simulink model "Quanser_AERO_Simulation_2020b"  (R2020b)
settings: Solver=ode45  StartTime=0.0  StopTime=sim_time  FixedStep=0.01  RelTol=1e-3
InitFcn:
  | % Run simulation parameters
  | quanser_AERO_sim_params;
model workspace (MAT data in the model file):
  a = Simulink.Parameter
  a.Value = 1.15
  a.DataType = 'auto'
  a.Dimensions = [1 1]
  a_a = Simulink.Parameter
  a_a.Value = 0.043381
  a_a.DataType = 'auto'
  a_a.Dimensions = [1 1]
  b = Simulink.Parameter
  b.Value = 0.2847
  b.DataType = 'auto'
  b.Dimensions = [1 1]
  b_b = Simulink.Parameter
  b_b.Value = 0.005
  b_b.DataType = 'auto'
  b_b.Dimensions = [1 1]
  c = Simulink.Parameter
  c.Value = 0.53573
  c.DataType = 'auto'
  c.Dimensions = [1 1]
  c_c = Simulink.Parameter
  c_c.Value = 0.005
  c_c.DataType = 'auto'
  c_c.Dimensions = [1 1]
  d = Simulink.Parameter
  d.Value = 0.0071058
  d.DataType = 'auto'
  d.Dimensions = [1 1]
  d_d = Simulink.Parameter
  d_d.Value = 0
  d_d.DataType = 'auto'
  d_d.Dimensions = [1 1]
  e = Simulink.Parameter
  e.Value = 0.0071
  e.DataType = 'auto'
  e.Dimensions = [1 1]
  f = Simulink.Parameter
  f.Value = 0.05
  f.DataType = 'auto'
  f.Dimensions = [1 1]
  g = Simulink.Parameter
  g.Value = 9.81
  g.DataType = 'auto'
  g.Dimensions = [1 1]
  p_p = Simulink.Parameter
  p_p.Value = 0.0005466
  p_p.DataType = 'auto'
  p_p.Dimensions = [1 1]
  smiData.RigidTransform(1).translation = [75 240 -4.4408920985e-15]
  smiData.RigidTransform(1).angle = 1.57079632679
  smiData.RigidTransform(1).axis = [5.55111512313e-17 1 5.55111512313e-17]
  smiData.RigidTransform(1).ID = 'B[AERO - Fork:1:-:AERO - Arm:1]'
  smiData.RigidTransform(2).translation = [0 0 72.5]
  smiData.RigidTransform(2).angle = 0
  smiData.RigidTransform(2).axis = [0 0 0]
  smiData.RigidTransform(2).ID = 'F[AERO - Fork:1:-:AERO - Arm:1]'
  smiData.RigidTransform(3).translation = [53 0 0]
  smiData.RigidTransform(3).angle = 1.57079632679
  smiData.RigidTransform(3).axis = [0 -1 0]
  smiData.RigidTransform(3).ID = 'B[AERO - Arm:1:-:AERO - Propeller Housing:1]'
  smiData.RigidTransform(4).translation = [-2.67952073108e-14 10 -95.5137103749]
  smiData.RigidTransform(4).angle = 3.14159265359
  smiData.RigidTransform(4).axis = [1 0 0]
  smiData.RigidTransform(4).ID = 'F[AERO - Arm:1:-:AERO - Propeller Housing:1]'
  smiData.RigidTransform(5).translation = [-53 0 0]
  smiData.RigidTransform(5).angle = 3.14159265359
  smiData.RigidTransform(5).axis = [0.707106781187 0 0.707106781187]
  smiData.RigidTransform(5).ID = 'B[AERO - Arm:1:-:AERO - Propeller Housing:2]'
  smiData.RigidTransform(6).translation = [-2.67952073108e-14 10 -95.5137103749]
  smiData.RigidTransform(6).angle = 3.14159265359
  smiData.RigidTransform(6).axis = [1 0 0]
  smiData.RigidTransform(6).ID = 'F[AERO - Arm:1:-:AERO - Propeller Housing:2]'
  smiData.RigidTransform(7).translation = [0 90 0]
  smiData.RigidTransform(7).angle = 2.09439510239
  smiData.RigidTransform(7).axis = [-0.57735026919 -0.57735026919 -0.57735026919]
  smiData.RigidTransform(7).ID = 'B[AERO - Base:1:-:AERO - Fork:1]'
  smiData.RigidTransform(8).translation = [0 -10 -1.83697019872e-15]
  smiData.RigidTransform(8).angle = 1.57079632679
  smiData.RigidTransform(8).axis = [-1 0 0]
  smiData.RigidTransform(8).ID = 'F[AERO - Base:1:-:AERO - Fork:1]'
  smiData.RigidTransform(9).translation = [0 7 0]
  smiData.RigidTransform(9).angle = 1.57079632679
  smiData.RigidTransform(9).axis = [-1 1.5327705937e-16 1.5327705937e-16]
  smiData.RigidTransform(9).ID = 'B[AERO - Propeller Housing:1:-:AERO - Propeller:1]'
  smiData.RigidTransform(10).translation = [0 2 0]
  smiData.RigidTransform(10).angle = 1.6664335536
  smiData.RigidTransform(10).axis = [-0.908660854566 0.295241808844 0.295241808844]
  smiData.RigidTransform(10).ID = 'F[AERO - Propeller Housing:1:-:AERO - Propeller:1]'
  smiData.RigidTransform(11).translation = [0 7 0]
  smiData.RigidTransform(11).angle = 1.57079632679
  smiData.RigidTransform(11).axis = [-1 6.25051204106e-17 6.25051204106e-17]
  smiData.RigidTransform(11).ID = 'B[AERO - Propeller Housing:2:-:AERO - Propeller:2]'
  smiData.RigidTransform(12).translation = [0 2 0]
  smiData.RigidTransform(12).angle = 2.28432867519
  smiData.RigidTransform(12).axis = [-0.456966311669 -0.628960169645 -0.628960169645]
  smiData.RigidTransform(12).ID = 'F[AERO - Propeller Housing:2:-:AERO - Propeller:2]'
  smiData.RigidTransform(13).translation = [-4.21383634609 -51.619496794 8.881784197e-15]
  smiData.RigidTransform(13).angle = 0
  smiData.RigidTransform(13).axis = [0 0 0]
  smiData.RigidTransform(13).ID = 'SixDofRigidTransform[AERO - Base:1]'
  smiData.Solid(1).mass = 2.36460135901
  smiData.Solid(1).CoM = [5.24111117378e-10 37.9532129776 0]
  smiData.Solid(1).MoI = [7187.732483 11870.3385044 7187.73246752]
  smiData.Solid(1).PoI = [0 0 -5.80827271444e-08]
  smiData.Solid(1).color = [0.0196078431373 0.0196078431373 0.0196078431373]
  smiData.Solid(1).opacity = 1
  smiData.Solid(1).ID = 'AERO - Base.ipt_{5B170AF7-4835-771C-6ADF-04BDBD784493}'
  smiData.Solid(2).mass = 0.833057949362
  smiData.Solid(2).CoM = [2.66169728603e-11 94.8876622043 1.47659785864e-12]
  smiData.Solid(2).MoI = [5303.1260885 5291.93963258 10383.1205417]
  smiData.Solid(2).PoI = [-1.78319566538e-10 1.20053300634e-10 2.21603950608e-09]
  smiData.Solid(2).color = [0.0196078431373 0.0196078431373 0.0196078431373]
  smiData.Solid(2).opacity = 1
  smiData.Solid(2).ID = 'AERO - Fork.ipt_{19DEB560-4DA8-F02E-E9C0-369FCF880C44}'
  smiData.Solid(3).mass = 0.268036846773
  smiData.Solid(3).CoM = [1.42171296006e-09 -5.19659809406e-10 0]
  smiData.Solid(3).MoI = [365.292105474 461.18513674 151.85502279]
  smiData.Solid(3).PoI = [9.09494701773e-14 -7.58518581279e-10 0]
  smiData.Solid(3).color = [0.0196078431373 0.0196078431373 0.0196078431373]
  smiData.Solid(3).opacity = 1
  smiData.Solid(3).ID = 'AERO - Arm.ipt_{15B1D815-460D-A329-2F9F-5FB9E93ED37B}'
  smiData.Solid(4).mass = 0.12383177107
  smiData.Solid(4).CoM = [0.00177195297055 5.45503898669 -8.60877968745]
  smiData.Solid(4).MoI = [310.701431452 411.715449483 138.600608927]
  smiData.Solid(4).PoI = [4.84491065682 -0.146839869659 -0.00100363322073]
  smiData.Solid(4).color = [0.0196078431373 0.0196078431373 0.0196078431373]
  smiData.Solid(4).opacity = 1
  smiData.Solid(4).ID = 'AERO - Propeller Housing.ipt_{180F9119-4C93-59E3-A88D-3BA97F46F3C3}'
  smiData.Solid(5).mass = 0.0206425497221
  smiData.Solid(5).CoM = [-1.0654070865e-12 5.09575570658 -2.10819251568e-11]
  smiData.Solid(5).MoI = [13.8216638961 27.2772869122 13.8216638974]
  smiData.Solid(5).PoI = [0 0 -9.39933149128e-14]
  smiData.Solid(5).color = [0.121568627451 0.121568627451 0.705882352941]
  smiData.Solid(5).opacity = 1
  smiData.Solid(5).ID = 'AERO - Propeller.ipt_{54ECD9B7-47A0-F6BB-CE8E-F5BB4731363E}'
  smiData.RevoluteJoint(1).Rz.Pos = 8.54433050095e-10
  smiData.RevoluteJoint(1).ID = '[AERO - Fork:1:-:AERO - Arm:1]'
  smiData.RevoluteJoint(2).Rz.Pos = 176.894023419
  smiData.RevoluteJoint(2).ID = '[AERO - Arm:1:-:AERO - Propeller Housing:1]'
  smiData.RevoluteJoint(3).Rz.Pos = 3.10597658118
  smiData.RevoluteJoint(3).ID = '[AERO - Arm:1:-:AERO - Propeller Housing:2]'
  smiData.RevoluteJoint(4).Rz.Pos = -4.73234748156e-11
  smiData.RevoluteJoint(4).ID = '[AERO - Base:1:-:AERO - Fork:1]'
  smiData.RevoluteJoint(5).Rz.Pos = -5.89066785065e-05
  smiData.RevoluteJoint(5).ID = '[AERO - Propeller Housing:1:-:AERO - Propeller:1]'
  smiData.RevoluteJoint(6).Rz.Pos = -3.64250166753e-05
  smiData.RevoluteJoint(6).ID = '[AERO - Propeller Housing:2:-:AERO - Propeller:2]'
  t_t = Simulink.Parameter
  t_t.Value = 0.0005466
  t_t.DataType = 'auto'
  t_t.Dimensions = [1 1]
  u_lim = Simulink.Parameter
  u_lim.Value = 24
  u_lim.DataType = 'auto'
  u_lim.Dimensions = [1 1]
  y_y = Simulink.Parameter
  y_y.Value = 0.02
  y_y.DataType = 'auto'
  y_y.Dimensions = [1 1]
  z_z = Simulink.Parameter
  z_z.Value = 0.01
  z_z.DataType = 'auto'
  z_z.Dimensions = [1 1]
undefined symbols (not defined in the file): A, A11, A12, A21, A22, A_tild, B, B1, B2, B_tild, C, C_tild, D_tild, ini_cond, Jr, KI, KII, KX, KXX, L, model, noise, ts, X, Y, Z
libraries: sm_lib x175, nesl_utility x35, simulink x30
(part 1 of 5)
settings Model: DataDictionary=AERO_DigitalTwin.sldd  OrderedModelArguments=off  Creator=garciar1  LastModifiedBy=linesLK

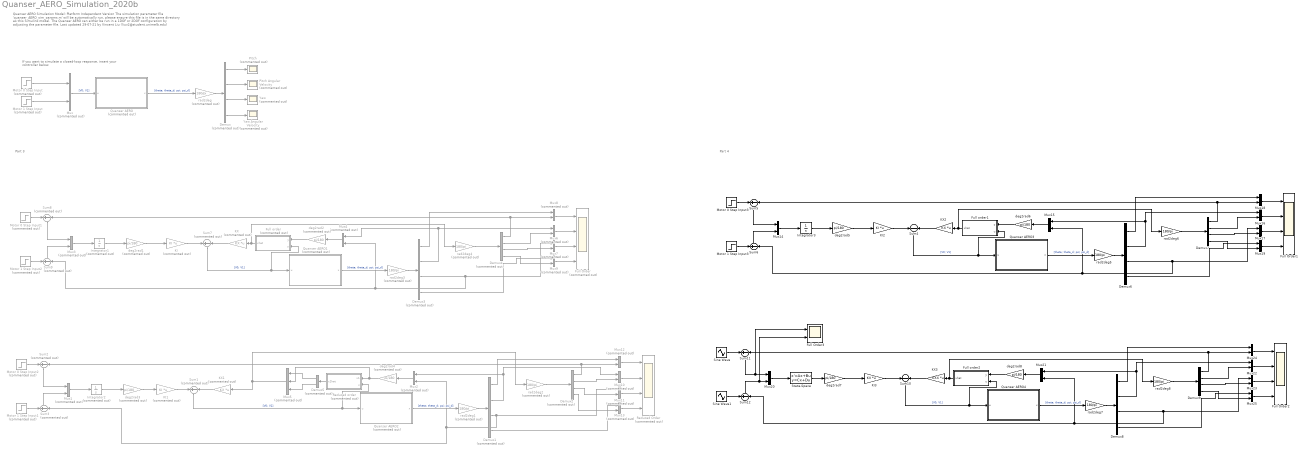
== system Quanser_AERO_Simulation_2020b ==
  note: If you want to simulate a closed-loop response, insert your controller below.
  note: Quanser AERO Simulation Model: Platform Independent Version
      | The simulation parameter file 'quanser_AERO_sim_params.m' will be automatically run, please ensure this file is in the same directory as this Simulink model. The Quanser AERO can either be run in a 1DOF or 2DOF configuration by adjusting the parameter file.
      | Last updated 29-07-21 by Vincent Liu (liuv2@student.unimelb.edu)
  note: Part 3
  note: Part 4
  Demux{,1..4} (5 alike) : Demux  Commented=on
  Demux5 : Demux  Commented=on  Outputs=2
  Demux{6..9} (4 alike) : Demux
  Full Order : Scope  Commented=on  NumInputPorts=4
  Full Order1 : Scope  NumInputPorts=4
  Full Order2 : Scope  NumInputPorts=4
  Full Order3 : Scope  NumInputPorts=2
  Full order : Subsystem  Commented=on
  Full order1 : Subsystem
  Full order2 : Subsystem
  Integrator1 : Integrator  Commented=on
  Integrator2 : Integrator  Commented=on
  Integrator3 : Integrator
  KI : Gain  Commented=on  Gain=KI  Multiplication=Matrix(K*u) (u vector)
  KI1 : Gain  Commented=on  Gain=KI  Multiplication=Matrix(K*u) (u vector)
  KI2 : Gain  Gain=KI  Multiplication=Matrix(K*u) (u vector)
  KI3 : Gain  Gain=KII  Multiplication=Matrix(K*u) (u vector)
  KX : Gain  Commented=on  Gain=KX  Multiplication=Matrix(K*u) (u vector)
  KX1 : Gain  Commented=on  Gain=KX  Multiplication=Matrix(K*u) (u vector)
  KX2 : Gain  Gain=KX  Multiplication=Matrix(K*u) (u vector)
  KX3 : Gain  Gain=KXX  Multiplication=Matrix(K*u) (u vector)
  Motor 0 Step Input : Step  Commented=on  After=20  SampleTime=0
  Motor 0 Step Input1 : Step  Commented=on  After=9  SampleTime=0
  Motor 0 Step Input2 : Step  Commented=on  After=9  SampleTime=0
  Motor 0 Step Input3 : Step  After=9  SampleTime=0
  Motor 1 Step Input : Step  Commented=on  After=10  SampleTime=0
  Motor 1 Step Input1 : Step  Commented=on  After=45  SampleTime=0
  Motor 1 Step Input2 : Step  Commented=on  After=45  SampleTime=0
  Motor 1 Step Input3 : Step  After=45  SampleTime=0
  Mux{,1..4,6..13} (13 alike) : Mux  Commented=on  Inputs=2
  Mux{14..25} (12 alike) : Mux  Inputs=2
  Mux5 : Mux  Commented=on  Inputs=3
  Pitch : Scope  Commented=on
  Pitch Angular Velocity : Scope  Commented=on
  Quanser AERO : Subsystem  Commented=on  TreatAsAtomicUnit=on
  Quanser AERO1 : Subsystem  Commented=on  TreatAsAtomicUnit=on
  Quanser AERO2 : Subsystem  Commented=on  TreatAsAtomicUnit=on
  Quanser AERO3 : Subsystem  TreatAsAtomicUnit=on
  Quanser AERO4 : Subsystem  TreatAsAtomicUnit=on
  Reduced Order : Scope  Commented=on  NumInputPorts=4
  Reduced order : Subsystem  Commented=on
  Sine Wave : Sin  Amplitude=9  Frequency=2*pi/5  SampleTime=0
  Sine Wave1 : Sin  Amplitude=30  Frequency=2*pi/5  SampleTime=0
  State-Space : StateSpace  A=A_tild  B=B_tild  C=C_tild  D=D_tild  InitialCondition=0
  Sum{1..3,7..9} (6 alike) : Sum  Commented=on  Inputs=+-
  Sum10 : Sum  Inputs=--
  Sum{5..6,11..12} (4 alike) : Sum  Inputs=+-
  Sum4 : Sum  Inputs=--
  Yaw : Scope  Commented=on
  Yaw Angular Velocity : Scope  Commented=on
  deg2rad{1..4} (4 alike) : Gain  Commented=on  Gain=pi/180
  deg2rad{5..8} (4 alike) : Gain  Gain=pi/180
  rad2deg{,1..4} (5 alike) : Gain  Commented=on  Gain=180/pi
  rad2deg{5..8} (4 alike) : Gain  Gain=180/pi
  wires:
  Demux/3 -> Yaw/1
  Demux/2 -> Pitch Angular Velocity/1
  Demux/4 -> Yaw Angular Velocity/1
  Mux/1 -> Quanser AERO/1(u)  "[V0; V1]"
  rad2deg/1 -> Demux/1
  Quanser AERO/1(x) -> rad2deg/1  "[theta; theta_d; psi; psi_d]"
  Motor 1 Step Input/1 -> Mux/2
  Motor 0 Step Input/1 -> Mux/1
  Demux/1 -> Pitch/1
  Mux3/1 -> Integrator1/1
  deg2rad1/1 -> KI/1
  Motor 1 Step Input2/1 -> Sum9/1
  Quanser AERO1/1(x) -> rad2deg3/1  "[theta; theta_d; psi; psi_d]"
  rad2deg3/1 -> Demux3/1
  KX/1 -> Sum7/2
  KI/1 -> Sum7/1
  Sum9/1 -> Mux3/2
  Sum7/1 -> Full order/2(u), Quanser AERO1/1(u)  "[V0; V1]"
  Integrator1/1 -> deg2rad1/1
  Motor 0 Step Input1/1 -> Sum8/1
  Sum8/1 -> Mux3/1
  Mux4/1 -> deg2rad2/1
  Full order/1(xhat) -> rad2deg4/1, KX/1
  deg2rad2/1 -> Full order/1(y)
  Demux4/3 -> Mux7/2
  rad2deg4/1 -> Demux4/1
  Demux3/2 -> Mux4/1, Mux6/1
  Demux4/2 -> Mux6/2
  Demux4/1 -> Mux8/2, Sum8/2
  Demux3/3 -> Mux7/1, Mux4/2, Sum9/2
  Sum2/1 -> Mux1/1
  KX1/1 -> Sum1/2
  Mux5/1 -> KX1/1, rad2deg2/1
  KI1/1 -> Sum1/1
  Quanser AERO2/1(x) -> rad2deg1/1  "[theta; theta_d; psi; psi_d]"
  Sum3/1 -> Mux1/2
  rad2deg2/1 -> Demux2/1
  Mux2/1 -> deg2rad4/1
  Motor 1 Step Input1/1 -> Sum3/1
  Motor 0 Step Input2/1 -> Sum2/1
  Sum1/1 -> Reduced order/2(u), Quanser AERO2/1(u)  "[V0; V1]"
  Demux1/3 -> Mux11/1, Mux2/2, Sum3/2
  Mux1/1 -> Integrator2/1
  deg2rad3/1 -> KI1/1
  Integrator2/1 -> deg2rad3/1
  rad2deg1/1 -> Demux1/1
  Demux2/1 -> Mux12/2, Sum2/2
  Demux1/2 -> Mux10/1, Mux2/1
  deg2rad4/1 -> Reduced order/1(x1), Mux5/2
  Reduced order/1(x2hat) -> Demux5/1
  Demux5/1 -> Mux5/1
  Demux5/2 -> Mux5/3
  Mux6/1 -> Full Order/2
  Mux7/1 -> Full Order/3
  Mux8/1 -> Full Order/1
  Demux3/1 -> Mux8/1
  Demux3/4 -> Mux9/1
  Demux4/4 -> Mux9/2
  Mux9/1 -> Full Order/4
  Mux13/1 -> Reduced Order/4
  Mux12/1 -> Reduced Order/1
  Mux11/1 -> Reduced Order/3
  Mux10/1 -> Reduced Order/2
  Demux1/1 -> Mux12/1
  Demux2/2 -> Mux10/2
  Demux2/3 -> Mux11/2
  Demux1/4 -> Mux13/1
  Demux2/4 -> Mux13/2
  deg2rad5/1 -> KI2/1
  Sum6/1 -> Mux14/2
  Demux7/4 -> Mux19/2
  Motor 0 Step Input3/1 -> Sum5/1
  Mux17/1 -> Full Order1/3
  Demux6/2 -> Mux16/1, Mux15/1
  Demux7/2 -> Mux16/2
  KI2/1 -> Sum4/1
  Quanser AERO3/1(x) -> rad2deg5/1  "[theta; theta_d; psi; psi_d]"
  KX2/1 -> Sum4/2
  deg2rad6/1 -> Full order1/1(y)
  Mux15/1 -> deg2rad6/1
  rad2deg6/1 -> Demux7/1
  Full order1/1(xhat) -> rad2deg6/1, KX2/1
  Demux6/1 -> Mux18/1
  rad2deg5/1 -> Demux6/1
  Sum4/1 -> Full order1/2(u), Quanser AERO3/1(u)  "[V0; V1]"
  Integrator3/1 -> deg2rad5/1
  Demux6/3 -> Mux17/1, Mux15/2, Sum6/2
  Mux14/1 -> Integrator3/1
  Mux18/1 -> Full Order1/1
  Motor 1 Step Input3/1 -> Sum6/1
  Mux16/1 -> Full Order1/2
  Sum5/1 -> Mux14/1
  Demux7/1 -> Mux18/2, Sum5/2
  Mux19/1 -> Full Order1/4
  Demux6/4 -> Mux19/1
  Demux7/3 -> Mux17/2
  Sum10/1 -> Full order2/2(u), Quanser AERO4/1(u)  "[V0; V1]"
  Sine Wave/1 -> Sum11/1
  Quanser AERO4/1(x) -> rad2deg7/1  "[theta; theta_d; psi; psi_d]"
  Demux9/3 -> Mux23/2
  deg2rad7/1 -> KI3/1
  rad2deg8/1 -> Demux9/1
  Demux9/4 -> Mux25/2
  Sum11/1 -> Full Order3/1, Mux20/1
  Mux20/1 -> State-Space/1
  KX3/1 -> Sum10/2
  Mux21/1 -> deg2rad8/1
  rad2deg7/1 -> Demux8/1
  Demux8/3 -> Mux23/1, Mux21/2, Sum12/2
  State-Space/1 -> deg2rad7/1
  deg2rad8/1 -> Full order2/1(y)
  Demux8/1 -> Mux24/1
  Sine Wave1/1 -> Sum12/1
  Demux8/2 -> Mux22/1, Mux21/1
  Mux22/1 -> Full Order2/2
  Mux24/1 -> Full Order2/1
  Demux9/1 -> Mux24/2, Sum11/2
  Mux25/1 -> Full Order2/4
  Demux9/2 -> Mux22/2
  Full order2/1(xhat) -> rad2deg8/1, KX3/1
  Demux8/4 -> Mux25/1
  Mux23/1 -> Full Order2/3
  KI3/1 -> Sum10/1
  Sum12/1 -> Full Order3/2, Mux20/2

== system Quanser_AERO_Simulation_2020b/Full order ==
  y : Inport
  u : Inport  Port=2
  A : Gain  Gain=A  Multiplication=Matrix(K*u) (u vector)
  B : Gain  Gain=B  Multiplication=Matrix(K*u) (u vector)
  C : Gain  Gain=C  Multiplication=Matrix(K*u) (u vector)
  Integrator1 : Integrator
  L : Gain  Gain=L  Multiplication=Matrix(K*u) (u vector)
  Sum1 : Sum  Inputs=+++
  Sum7 : Sum  Inputs=+-
  xhat : Outport
  wires:
  u/1 -> B/1
  Sum1/1 -> Integrator1/1
  y/1 -> Sum7/1
  C/1 -> Sum7/2
  Sum7/1 -> L/1
  L/1 -> Sum1/1
  B/1 -> Sum1/2
  A/1 -> Sum1/3
  Integrator1/1 -> C/1, A/1, xhat/1

== system Quanser_AERO_Simulation_2020b/Full order1 ==
  y : Inport
  u : Inport  Port=2
  A : Gain  Gain=A  Multiplication=Matrix(K*u) (u vector)
  B : Gain  Gain=B  Multiplication=Matrix(K*u) (u vector)
  C : Gain  Gain=C  Multiplication=Matrix(K*u) (u vector)
  Integrator1 : Integrator
  L : Gain  Gain=L  Multiplication=Matrix(K*u) (u vector)
  Sum1 : Sum  Inputs=+++
  Sum7 : Sum  Inputs=+-
  xhat : Outport
  wires:
  u/1 -> B/1
  Sum1/1 -> Integrator1/1
  y/1 -> Sum7/1
  C/1 -> Sum7/2
  Sum7/1 -> L/1
  L/1 -> Sum1/1
  B/1 -> Sum1/2
  A/1 -> Sum1/3
  Integrator1/1 -> C/1, A/1, xhat/1

== system Quanser_AERO_Simulation_2020b/Full order2 ==
  y : Inport
  u : Inport  Port=2
  A : Gain  Gain=A  Multiplication=Matrix(K*u) (u vector)
  B : Gain  Gain=B  Multiplication=Matrix(K*u) (u vector)
  C : Gain  Gain=C  Multiplication=Matrix(K*u) (u vector)
  Integrator1 : Integrator
  L : Gain  Gain=L  Multiplication=Matrix(K*u) (u vector)
  Sum1 : Sum  Inputs=+++
  Sum7 : Sum  Inputs=+-
  xhat : Outport
  wires:
  u/1 -> B/1
  Sum1/1 -> Integrator1/1
  y/1 -> Sum7/1
  C/1 -> Sum7/2
  Sum7/1 -> L/1
  L/1 -> Sum1/1
  B/1 -> Sum1/2
  A/1 -> Sum1/3
  Integrator1/1 -> C/1, A/1, xhat/1

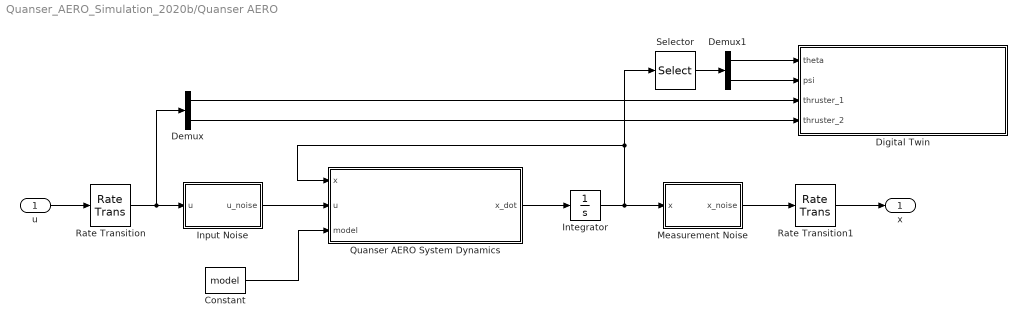
== system Quanser_AERO_Simulation_2020b/Quanser AERO ==
  u : Inport
  Constant : Constant  Value=model
  Demux : Demux  Outputs=2
  Demux1 : Demux  Outputs=2
  Digital Twin : Subsystem
  Input Noise : Subsystem  TreatAsAtomicUnit=on
  Integrator : Integrator  InitialCondition=[ini_cond.theta; ini_cond.theta_dot; ini_cond.psi; ini_cond.psi_dot]
  Measurement Noise : Subsystem  TreatAsAtomicUnit=on
  Quanser AERO System Dynamics : Subsystem  TreatAsAtomicUnit=on
  Rate Transition : RateTransition  OutPortSampleTime=ts
  Rate Transition1 : RateTransition  InitialCondition=[ini_cond.theta; ini_cond.theta_dot; ini_cond.psi; ini_cond.psi_dot]  OutPortSampleTime=ts
  Selector : Selector  InputPortWidth=4  IndexOptions=Index vector (dialog)  Indices=[1 3]  OutputSizes=1
  x : Outport  VectorParamsAs1DForOutWhenUnconnected=off
  wires:
  u/1 -> Rate Transition/1
  Rate Transition/1 -> Input Noise/1(u), Demux/1
  Rate Transition1/1 -> x/1
  Input Noise/1(u_noise) -> Quanser AERO System Dynamics/2(u)
  Measurement Noise/1(x_noise) -> Rate Transition1/1
  Selector/1 -> Demux1/1
  Demux/1 -> Digital Twin/3(thruster_1)
  Demux/2 -> Digital Twin/4(thruster_2)
  Demux1/1 -> Digital Twin/1(theta)
  Demux1/2 -> Digital Twin/2(psi)
  Integrator/1 -> Measurement Noise/1(x), Selector/1, Quanser AERO System Dynamics/1(x)
  Constant/1 -> Quanser AERO System Dynamics/3(model)
  Quanser AERO System Dynamics/1(x_dot) -> Integrator/1

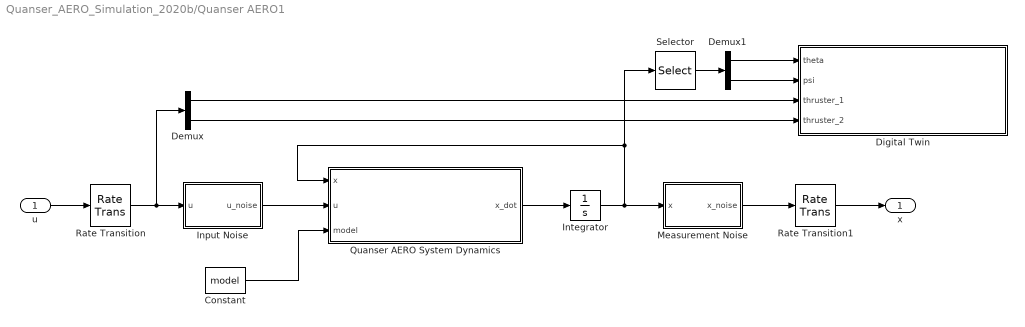
== system Quanser_AERO_Simulation_2020b/Quanser AERO1 ==
  u : Inport
  Constant : Constant  Value=model
  Demux : Demux  Outputs=2
  Demux1 : Demux  Outputs=2
  Digital Twin : Subsystem
  Input Noise : Subsystem  TreatAsAtomicUnit=on
  Integrator : Integrator  InitialCondition=[ini_cond.theta; ini_cond.theta_dot; ini_cond.psi; ini_cond.psi_dot]
  Measurement Noise : Subsystem  TreatAsAtomicUnit=on
  Quanser AERO System Dynamics : Subsystem  TreatAsAtomicUnit=on
  Rate Transition : RateTransition  OutPortSampleTime=ts
  Rate Transition1 : RateTransition  InitialCondition=[ini_cond.theta; ini_cond.theta_dot; ini_cond.psi; ini_cond.psi_dot]  OutPortSampleTime=ts
  Selector : Selector  InputPortWidth=4  IndexOptions=Index vector (dialog)  Indices=[1 3]  OutputSizes=1
  x : Outport  VectorParamsAs1DForOutWhenUnconnected=off
  wires:
  u/1 -> Rate Transition/1
  Rate Transition/1 -> Input Noise/1(u), Demux/1
  Rate Transition1/1 -> x/1
  Input Noise/1(u_noise) -> Quanser AERO System Dynamics/2(u)
  Measurement Noise/1(x_noise) -> Rate Transition1/1
  Selector/1 -> Demux1/1
  Demux/1 -> Digital Twin/3(thruster_1)
  Demux/2 -> Digital Twin/4(thruster_2)
  Demux1/1 -> Digital Twin/1(theta)
  Demux1/2 -> Digital Twin/2(psi)
  Integrator/1 -> Measurement Noise/1(x), Selector/1, Quanser AERO System Dynamics/1(x)
  Constant/1 -> Quanser AERO System Dynamics/3(model)
  Quanser AERO System Dynamics/1(x_dot) -> Integrator/1

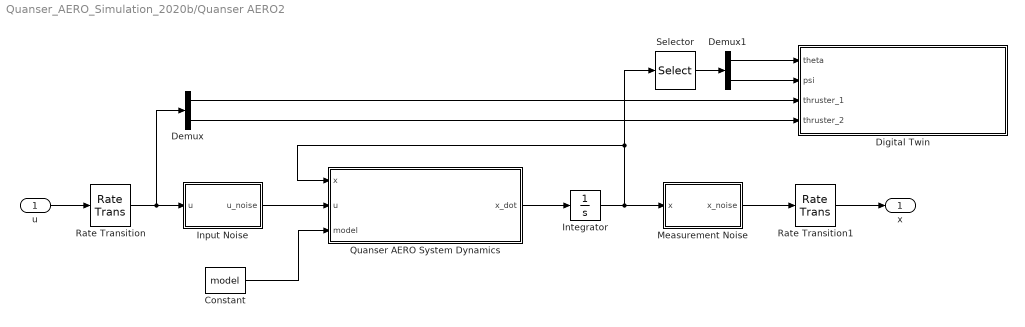
== system Quanser_AERO_Simulation_2020b/Quanser AERO2 ==
  u : Inport
  Constant : Constant  Value=model
  Demux : Demux  Outputs=2
  Demux1 : Demux  Outputs=2
  Digital Twin : Subsystem
  Input Noise : Subsystem  TreatAsAtomicUnit=on
  Integrator : Integrator  InitialCondition=[ini_cond.theta; ini_cond.theta_dot; ini_cond.psi; ini_cond.psi_dot]
  Measurement Noise : Subsystem  TreatAsAtomicUnit=on
  Quanser AERO System Dynamics : Subsystem  TreatAsAtomicUnit=on
  Rate Transition : RateTransition  OutPortSampleTime=ts
  Rate Transition1 : RateTransition  InitialCondition=[ini_cond.theta; ini_cond.theta_dot; ini_cond.psi; ini_cond.psi_dot]  OutPortSampleTime=ts
  Selector : Selector  InputPortWidth=4  IndexOptions=Index vector (dialog)  Indices=[1 3]  OutputSizes=1
  x : Outport  VectorParamsAs1DForOutWhenUnconnected=off
  wires:
  u/1 -> Rate Transition/1
  Rate Transition/1 -> Input Noise/1(u), Demux/1
  Rate Transition1/1 -> x/1
  Input Noise/1(u_noise) -> Quanser AERO System Dynamics/2(u)
  Measurement Noise/1(x_noise) -> Rate Transition1/1
  Selector/1 -> Demux1/1
  Demux/1 -> Digital Twin/3(thruster_1)
  Demux/2 -> Digital Twin/4(thruster_2)
  Demux1/1 -> Digital Twin/1(theta)
  Demux1/2 -> Digital Twin/2(psi)
  Integrator/1 -> Measurement Noise/1(x), Selector/1, Quanser AERO System Dynamics/1(x)
  Constant/1 -> Quanser AERO System Dynamics/3(model)
  Quanser AERO System Dynamics/1(x_dot) -> Integrator/1

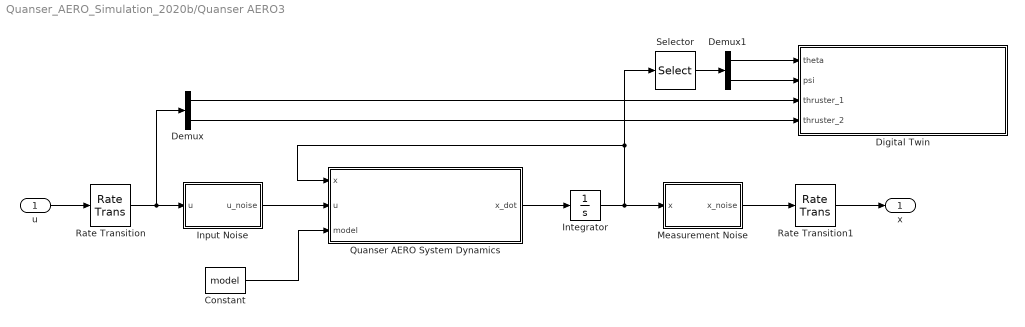
== system Quanser_AERO_Simulation_2020b/Quanser AERO3 ==
  u : Inport
  Constant : Constant  Value=model
  Demux : Demux  Outputs=2
  Demux1 : Demux  Outputs=2
  Digital Twin : Subsystem
  Input Noise : Subsystem  TreatAsAtomicUnit=on
  Integrator : Integrator  InitialCondition=[ini_cond.theta; ini_cond.theta_dot; ini_cond.psi; ini_cond.psi_dot]
  Measurement Noise : Subsystem  TreatAsAtomicUnit=on
  Quanser AERO System Dynamics : Subsystem  TreatAsAtomicUnit=on
  Rate Transition : RateTransition  OutPortSampleTime=ts
  Rate Transition1 : RateTransition  InitialCondition=[ini_cond.theta; ini_cond.theta_dot; ini_cond.psi; ini_cond.psi_dot]  OutPortSampleTime=ts
  Selector : Selector  InputPortWidth=4  IndexOptions=Index vector (dialog)  Indices=[1 3]  OutputSizes=1
  x : Outport  VectorParamsAs1DForOutWhenUnconnected=off
  wires:
  u/1 -> Rate Transition/1
  Rate Transition/1 -> Input Noise/1(u), Demux/1
  Rate Transition1/1 -> x/1
  Input Noise/1(u_noise) -> Quanser AERO System Dynamics/2(u)
  Measurement Noise/1(x_noise) -> Rate Transition1/1
  Selector/1 -> Demux1/1
  Demux/1 -> Digital Twin/3(thruster_1)
  Demux/2 -> Digital Twin/4(thruster_2)
  Demux1/1 -> Digital Twin/1(theta)
  Demux1/2 -> Digital Twin/2(psi)
  Integrator/1 -> Measurement Noise/1(x), Selector/1, Quanser AERO System Dynamics/1(x)
  Constant/1 -> Quanser AERO System Dynamics/3(model)
  Quanser AERO System Dynamics/1(x_dot) -> Integrator/1

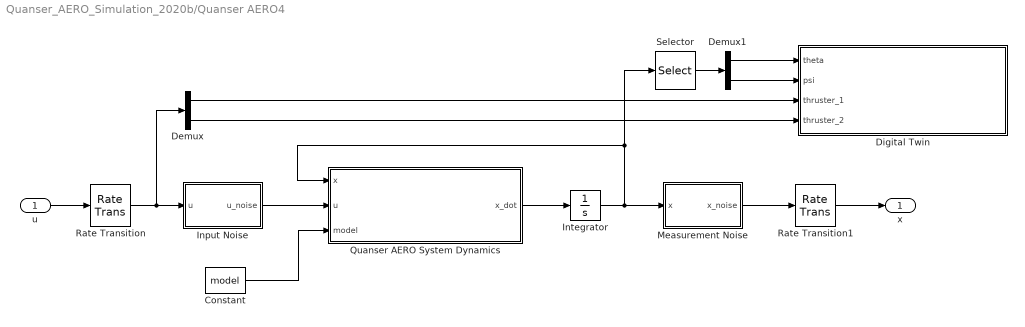
== system Quanser_AERO_Simulation_2020b/Quanser AERO4 ==
  u : Inport
  Constant : Constant  Value=model
  Demux : Demux  Outputs=2
  Demux1 : Demux  Outputs=2
  Digital Twin : Subsystem
  Input Noise : Subsystem  TreatAsAtomicUnit=on
  Integrator : Integrator  InitialCondition=[ini_cond.theta; ini_cond.theta_dot; ini_cond.psi; ini_cond.psi_dot]
  Measurement Noise : Subsystem  TreatAsAtomicUnit=on
  Quanser AERO System Dynamics : Subsystem  TreatAsAtomicUnit=on
  Rate Transition : RateTransition  OutPortSampleTime=ts
  Rate Transition1 : RateTransition  InitialCondition=[ini_cond.theta; ini_cond.theta_dot; ini_cond.psi; ini_cond.psi_dot]  OutPortSampleTime=ts
  Selector : Selector  InputPortWidth=4  IndexOptions=Index vector (dialog)  Indices=[1 3]  OutputSizes=1
  x : Outport  VectorParamsAs1DForOutWhenUnconnected=off
  wires:
  u/1 -> Rate Transition/1
  Rate Transition/1 -> Input Noise/1(u), Demux/1
  Rate Transition1/1 -> x/1
  Input Noise/1(u_noise) -> Quanser AERO System Dynamics/2(u)
  Measurement Noise/1(x_noise) -> Rate Transition1/1
  Selector/1 -> Demux1/1
  Demux/1 -> Digital Twin/3(thruster_1)
  Demux/2 -> Digital Twin/4(thruster_2)
  Demux1/1 -> Digital Twin/1(theta)
  Demux1/2 -> Digital Twin/2(psi)
  Integrator/1 -> Measurement Noise/1(x), Selector/1, Quanser AERO System Dynamics/1(x)
  Constant/1 -> Quanser AERO System Dynamics/3(model)
  Quanser AERO System Dynamics/1(x_dot) -> Integrator/1

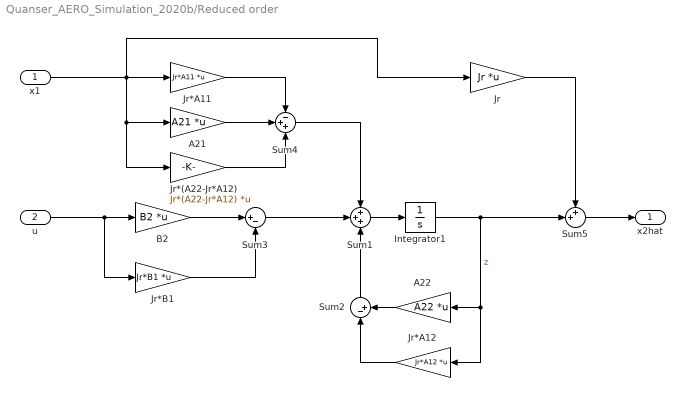
== system Quanser_AERO_Simulation_2020b/Reduced order ==
  x1 : Inport
  u : Inport  Port=2
  A21 : Gain  Gain=A21  Multiplication=Matrix(K*u) (u vector)
  A22 : Gain  Gain=A22  Multiplication=Matrix(K*u) (u vector)
  B2 : Gain  Gain=B2  Multiplication=Matrix(K*u) (u vector)
  Integrator1 : Integrator
  Jr : Gain  Gain=Jr  Multiplication=Matrix(K*u) (u vector)
  Jr*(A22-Jr*A12) : Gain  Gain=Jr*(A22-Jr*A12)  Multiplication=Matrix(K*u) (u vector)
  Jr*A11 : Gain  Gain=Jr*A11  Multiplication=Matrix(K*u) (u vector)
  Jr*A12 : Gain  Gain=Jr*A12  Multiplication=Matrix(K*u) (u vector)
  Jr*B1 : Gain  Gain=Jr*B1  Multiplication=Matrix(K*u) (u vector)
  Sum1 : Sum  Inputs=+++
  Sum2 : Sum  Inputs=|-+
  Sum3 : Sum  Inputs=|+-
  Sum4 : Sum  Inputs=-++
  Sum5 : Sum  Inputs=++|
  x2hat : Outport
  wires:
  Jr/1 -> Sum5/1
  B2/1 -> Sum3/1
  Sum4/1 -> Sum1/1
  Sum1/1 -> Integrator1/1
  Sum5/1 -> x2hat/1
  Sum2/1 -> Sum1/3
  Integrator1/1 -> Sum5/2, Jr*A12/1, A22/1  "z"
  Jr*A12/1 -> Sum2/1
  A21/1 -> Sum4/2
  Jr*A11/1 -> Sum4/1
  A22/1 -> Sum2/2
  x1/1 -> Jr*(A22-Jr*A12)/1, A21/1, Jr/1, Jr*A11/1
  u/1 -> Jr*B1/1, B2/1
  Jr*B1/1 -> Sum3/2
  Sum3/1 -> Sum1/2
  Jr*(A22-Jr*A12)/1 -> Sum4/3

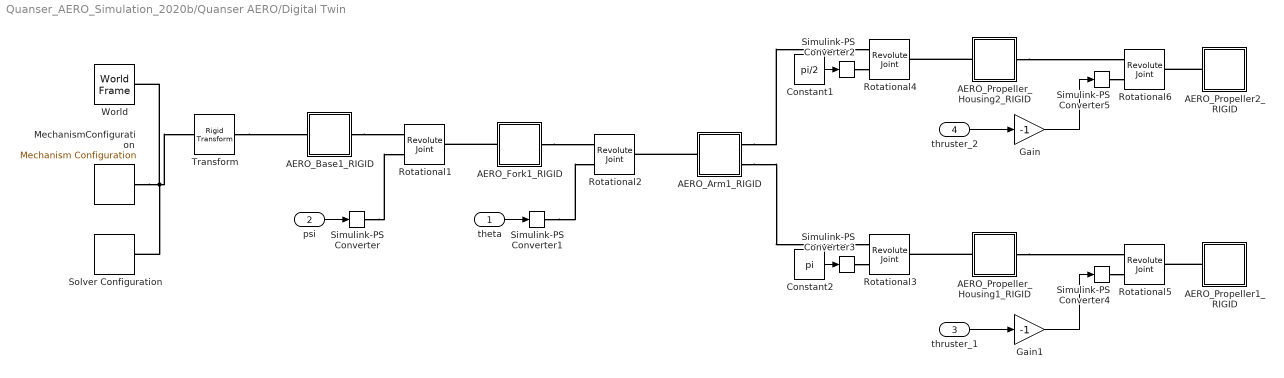
== system Quanser_AERO_Simulation_2020b/Quanser AERO/Digital Twin ==
  theta : Inport
  psi : Inport  Port=2
  thruster_1 : Inport  Port=3
  thruster_2 : Inport  Port=4
  AERO_Arm1_RIGID : Subsystem
  AERO_Base1_RIGID : Subsystem
  AERO_Fork1_RIGID : Subsystem
  AERO_Propeller1_RIGID : Subsystem
  AERO_Propeller2_RIGID : Subsystem
  AERO_Propeller_Housing1_RIGID : Subsystem
  AERO_Propeller_Housing2_RIGID : Subsystem
  Constant1 : Constant  Value=pi/2
  Constant2 : Constant  Value=pi
  Gain : Gain  Gain=-1
  Gain1 : Gain  Gain=-1
  MechanismConfiguration : sm_lib/Utilities/Mechanism Configuration  UniformGravity=Constant  GravityVector=[0 -9.80665 0]  GravityVectorUnits=m/s^2  GravityUnits=m/s^2  LinearizationDelta=0.001  JointModeTransitionNonlinearIterations=2
  Rotational1 : sm_lib/Joints/Revolute Joint  JointMode=Normal  SenseConstraintForce=off  SenseConstraintForceX=off  SenseConstraintForceY=off  SenseConstraintForceZ=off  SenseConstraintTorque=off  SenseConstraintTorqueX=off  SenseConstraintTorqueY=off  SenseConstraintTorqueZ=off  SenseTotalForce=off  SenseTotalForceX=off  SenseTotalForceY=off  SenseTotalForceZ=off  SenseTotalTorque=off  SenseTotalTorqueX=off  SenseTotalTorqueY=off  SenseTotalTorqueZ=off  CompositeWrenchDir=FollowerOnBase  CompositeWrenchFrame=BaseFrame  EquilibriumPosition=0  EquilibriumPositionUnits=deg  SpringStiffness=0  SpringStiffnessUnits=N*m/deg  DampingCoefficient=0  DampingCoefficientUnits=N*m/(deg/s)  TorqueActuationMode=ComputedTorque  MotionActuationMode=InputMotion  SensePosition=off  SenseVelocity=off  SenseAcceleration=off  SenseTorqueForce=off  SenseLowerLimitTorqueForce=off  SenseUpperLimitTorqueForce=off  LowerLimitSpecify=off  LowerLimitBound=-90  LowerLimitBoundUnits=deg  LowerLimitStiffness=1e4  LowerLimitStiffnessUnits=N*m/deg  LowerLimitDamping=10  LowerLimitDampingUnits=N*m/(deg/s)  LowerLimitTransitionRegionWidth=0.1  LowerLimitTransitionRegionWidthUnits=deg  UpperLimitSpecify=off  UpperLimitBound=90  UpperLimitBoundUnits=deg  UpperLimitStiffness=1e4  UpperLimitStiffnessUnits=N*m/deg  UpperLimitDamping=10  UpperLimitDampingUnits=N*m/(deg/s)  UpperLimitTransitionRegionWidth=0.1  UpperLimitTransitionRegionWidthUnits=deg  PositionTargetSpecify=on  PositionTargetPriority=Low  PositionTargetValue=smiData.RevoluteJoint(4).Rz.Pos  PositionTargetValueUnits=deg  VelocityTargetSpecify=off  VelocityTargetPriority=High  VelocityTargetValue=0  VelocityTargetValueUnits=deg/s
  Rotational2 : sm_lib/Joints/Revolute Joint  JointMode=Normal  SenseConstraintForce=off  SenseConstraintForceX=off  SenseConstraintForceY=off  SenseConstraintForceZ=off  SenseConstraintTorque=off  SenseConstraintTorqueX=off  SenseConstraintTorqueY=off  SenseConstraintTorqueZ=off  SenseTotalForce=off  SenseTotalForceX=off  SenseTotalForceY=off  SenseTotalForceZ=off  SenseTotalTorque=off  SenseTotalTorqueX=off  SenseTotalTorqueY=off  SenseTotalTorqueZ=off  CompositeWrenchDir=FollowerOnBase  CompositeWrenchFrame=BaseFrame  EquilibriumPosition=0  EquilibriumPositionUnits=deg  SpringStiffness=0  SpringStiffnessUnits=N*m/deg  DampingCoefficient=0  DampingCoefficientUnits=N*m/(deg/s)  TorqueActuationMode=ComputedTorque  MotionActuationMode=InputMotion  SensePosition=off  SenseVelocity=off  SenseAcceleration=off  SenseTorqueForce=off  SenseLowerLimitTorqueForce=off  SenseUpperLimitTorqueForce=off  LowerLimitSpecify=off  LowerLimitBound=-90  LowerLimitBoundUnits=deg  LowerLimitStiffness=1e4  LowerLimitStiffnessUnits=N*m/deg  LowerLimitDamping=10  LowerLimitDampingUnits=N*m/(deg/s)  LowerLimitTransitionRegionWidth=0.1  LowerLimitTransitionRegionWidthUnits=deg  UpperLimitSpecify=off  UpperLimitBound=90  UpperLimitBoundUnits=deg  UpperLimitStiffness=1e4  UpperLimitStiffnessUnits=N*m/deg  UpperLimitDamping=10  UpperLimitDampingUnits=N*m/(deg/s)  UpperLimitTransitionRegionWidth=0.1  UpperLimitTransitionRegionWidthUnits=deg  PositionTargetSpecify=on  PositionTargetPriority=Low  PositionTargetValue=smiData.RevoluteJoint(1).Rz.Pos  PositionTargetValueUnits=deg  VelocityTargetSpecify=off  VelocityTargetPriority=High  VelocityTargetValue=0  VelocityTargetValueUnits=deg/s
  Rotational3 : sm_lib/Joints/Revolute Joint  JointMode=Normal  SenseConstraintForce=off  SenseConstraintForceX=off  SenseConstraintForceY=off  SenseConstraintForceZ=off  SenseConstraintTorque=off  SenseConstraintTorqueX=off  SenseConstraintTorqueY=off  SenseConstraintTorqueZ=off  SenseTotalForce=off  SenseTotalForceX=off  SenseTotalForceY=off  SenseTotalForceZ=off  SenseTotalTorque=off  SenseTotalTorqueX=off  SenseTotalTorqueY=off  SenseTotalTorqueZ=off  CompositeWrenchDir=FollowerOnBase  CompositeWrenchFrame=BaseFrame  EquilibriumPosition=0  EquilibriumPositionUnits=deg  SpringStiffness=0  SpringStiffnessUnits=N*m/deg  DampingCoefficient=0  DampingCoefficientUnits=N*m/(deg/s)  TorqueActuationMode=ComputedTorque  MotionActuationMode=InputMotion  SensePosition=off  SenseVelocity=off  SenseAcceleration=off  SenseTorqueForce=off  SenseLowerLimitTorqueForce=off  SenseUpperLimitTorqueForce=off  LowerLimitSpecify=off  LowerLimitBound=-90  LowerLimitBoundUnits=deg  LowerLimitStiffness=1e4  LowerLimitStiffnessUnits=N*m/deg  LowerLimitDamping=10  LowerLimitDampingUnits=N*m/(deg/s)  LowerLimitTransitionRegionWidth=0.1  LowerLimitTransitionRegionWidthUnits=deg  UpperLimitSpecify=off  UpperLimitBound=90  UpperLimitBoundUnits=deg  UpperLimitStiffness=1e4  UpperLimitStiffnessUnits=N*m/deg  UpperLimitDamping=10  UpperLimitDampingUnits=N*m/(deg/s)  UpperLimitTransitionRegionWidth=0.1  UpperLimitTransitionRegionWidthUnits=deg  PositionTargetSpecify=on  PositionTargetPriority=High  PositionTargetValue=smiData.RevoluteJoint(2).Rz.Pos  PositionTargetValueUnits=deg  VelocityTargetSpecify=off  VelocityTargetPriority=High  VelocityTargetValue=0  VelocityTargetValueUnits=deg/s
  Rotational4 : sm_lib/Joints/Revolute Joint  JointMode=Normal  SenseConstraintForce=off  SenseConstraintForceX=off  SenseConstraintForceY=off  SenseConstraintForceZ=off  SenseConstraintTorque=off  SenseConstraintTorqueX=off  SenseConstraintTorqueY=off  SenseConstraintTorqueZ=off  SenseTotalForce=off  SenseTotalForceX=off  SenseTotalForceY=off  SenseTotalForceZ=off  SenseTotalTorque=off  SenseTotalTorqueX=off  SenseTotalTorqueY=off  SenseTotalTorqueZ=off  CompositeWrenchDir=FollowerOnBase  CompositeWrenchFrame=BaseFrame  EquilibriumPosition=0  EquilibriumPositionUnits=deg  SpringStiffness=0  SpringStiffnessUnits=N*m/deg  DampingCoefficient=0  DampingCoefficientUnits=N*m/(deg/s)  TorqueActuationMode=ComputedTorque  MotionActuationMode=InputMotion  SensePosition=off  SenseVelocity=off  SenseAcceleration=off  SenseTorqueForce=off  SenseLowerLimitTorqueForce=off  SenseUpperLimitTorqueForce=off  LowerLimitSpecify=off  LowerLimitBound=-90  LowerLimitBoundUnits=deg  LowerLimitStiffness=1e4  LowerLimitStiffnessUnits=N*m/deg  LowerLimitDamping=10  LowerLimitDampingUnits=N*m/(deg/s)  LowerLimitTransitionRegionWidth=0.1  LowerLimitTransitionRegionWidthUnits=deg  UpperLimitSpecify=off  UpperLimitBound=90  UpperLimitBoundUnits=deg  UpperLimitStiffness=1e4  UpperLimitStiffnessUnits=N*m/deg  UpperLimitDamping=10  UpperLimitDampingUnits=N*m/(deg/s)  UpperLimitTransitionRegionWidth=0.1  UpperLimitTransitionRegionWidthUnits=deg  PositionTargetSpecify=on  PositionTargetPriority=Low  PositionTargetValue=smiData.RevoluteJoint(3).Rz.Pos  PositionTargetValueUnits=deg  VelocityTargetSpecify=off  VelocityTargetPriority=High  VelocityTargetValue=0  VelocityTargetValueUnits=deg/s
  Rotational5 : sm_lib/Joints/Revolute Joint  JointMode=Normal  SenseConstraintForce=off  SenseConstraintForceX=off  SenseConstraintForceY=off  SenseConstraintForceZ=off  SenseConstraintTorque=off  SenseConstraintTorqueX=off  SenseConstraintTorqueY=off  SenseConstraintTorqueZ=off  SenseTotalForce=off  SenseTotalForceX=off  SenseTotalForceY=off  SenseTotalForceZ=off  SenseTotalTorque=off  SenseTotalTorqueX=off  SenseTotalTorqueY=off  SenseTotalTorqueZ=off  CompositeWrenchDir=FollowerOnBase  CompositeWrenchFrame=BaseFrame  EquilibriumPosition=0  EquilibriumPositionUnits=deg  SpringStiffness=0  SpringStiffnessUnits=N*m/deg  DampingCoefficient=0.000001  DampingCoefficientUnits=N*m/(deg/s)  TorqueActuationMode=InputTorque  MotionActuationMode=ComputedMotion  SensePosition=off  SenseVelocity=off  SenseAcceleration=off  SenseTorqueForce=off  SenseLowerLimitTorqueForce=off  SenseUpperLimitTorqueForce=off  LowerLimitSpecify=off  LowerLimitBound=-90  LowerLimitBoundUnits=deg  LowerLimitStiffness=1e4  LowerLimitStiffnessUnits=N*m/deg  LowerLimitDamping=10  LowerLimitDampingUnits=N*m/(deg/s)  LowerLimitTransitionRegionWidth=0.1  LowerLimitTransitionRegionWidthUnits=deg  UpperLimitSpecify=off  UpperLimitBound=90  UpperLimitBoundUnits=deg  UpperLimitStiffness=1e4  UpperLimitStiffnessUnits=N*m/deg  UpperLimitDamping=10  UpperLimitDampingUnits=N*m/(deg/s)  UpperLimitTransitionRegionWidth=0.1  UpperLimitTransitionRegionWidthUnits=deg  PositionTargetSpecify=on  PositionTargetPriority=Low  PositionTargetValue=smiData.RevoluteJoint(5).Rz.Pos  PositionTargetValueUnits=deg  VelocityTargetSpecify=off  VelocityTargetPriority=High  VelocityTargetValue=0  VelocityTargetValueUnits=deg/s
  Rotational6 : sm_lib/Joints/Revolute Joint  JointMode=Normal  SenseConstraintForce=off  SenseConstraintForceX=off  SenseConstraintForceY=off  SenseConstraintForceZ=off  SenseConstraintTorque=off  SenseConstraintTorqueX=off  SenseConstraintTorqueY=off  SenseConstraintTorqueZ=off  SenseTotalForce=off  SenseTotalForceX=off  SenseTotalForceY=off  SenseTotalForceZ=off  SenseTotalTorque=off  SenseTotalTorqueX=off  SenseTotalTorqueY=off  SenseTotalTorqueZ=off  CompositeWrenchDir=FollowerOnBase  CompositeWrenchFrame=BaseFrame  EquilibriumPosition=0  EquilibriumPositionUnits=deg  SpringStiffness=0  SpringStiffnessUnits=N*m/deg  DampingCoefficient=0.000001  DampingCoefficientUnits=N*m/(rad/s)  TorqueActuationMode=InputTorque  MotionActuationMode=ComputedMotion  SensePosition=off  SenseVelocity=off  SenseAcceleration=off  SenseTorqueForce=off  SenseLowerLimitTorqueForce=off  SenseUpperLimitTorqueForce=off  LowerLimitSpecify=off  LowerLimitBound=-90  LowerLimitBoundUnits=deg  LowerLimitStiffness=1e4  LowerLimitStiffnessUnits=N*m/deg  LowerLimitDamping=10  LowerLimitDampingUnits=N*m/(deg/s)  LowerLimitTransitionRegionWidth=0.1  LowerLimitTransitionRegionWidthUnits=deg  UpperLimitSpecify=off  UpperLimitBound=90  UpperLimitBoundUnits=deg  UpperLimitStiffness=1e4  UpperLimitStiffnessUnits=N*m/deg  UpperLimitDamping=10  UpperLimitDampingUnits=N*m/(deg/s)  UpperLimitTransitionRegionWidth=0.1  UpperLimitTransitionRegionWidthUnits=deg  PositionTargetSpecify=on  PositionTargetPriority=Low  PositionTargetValue=smiData.RevoluteJoint(6).Rz.Pos  PositionTargetValueUnits=deg  VelocityTargetSpecify=off  VelocityTargetPriority=High  VelocityTargetValue=0  VelocityTargetValueUnits=deg/s
  Simulink-PS Converter{,1..3} (4 alike) : nesl_utility/Simulink-PS Converter  PhysicalDomain=network_engine_domain  SubClassName=ps_input  LeftPortType=input  RightPortType=output  PseudoPeriodic=off  Frequencies=[]  NoiseDistribution=none  NoiseParameters=[]  Unit=1  AffineConversion=off  FilteringAndDerivatives=filter  SimscapeFilterOrder=2  InputFilterTimeConstant=0.001  UdotUserProvided=0
      settings: SourceProductBaseCode=PW,SS
  Simulink-PS Converter4 : nesl_utility/Simulink-PS Converter  PhysicalDomain=network_engine_domain  SubClassName=ps_input  LeftPortType=input  RightPortType=output  PseudoPeriodic=off  Frequencies=[]  NoiseDistribution=none  NoiseParameters=[]  Unit=1  AffineConversion=off  FilteringAndDerivatives=provide  SimscapeFilterOrder=2  InputFilterTimeConstant=0.001  UdotUserProvided=0
      settings: SourceProductBaseCode=PW,SS
  Simulink-PS Converter5 : nesl_utility/Simulink-PS Converter  PhysicalDomain=network_engine_domain  SubClassName=ps_input  LeftPortType=input  RightPortType=output  PseudoPeriodic=off  Frequencies=[]  NoiseDistribution=none  NoiseParameters=[]  Unit=1  AffineConversion=off  FilteringAndDerivatives=provide  SimscapeFilterOrder=2  InputFilterTimeConstant=0.001  UdotUserProvided=0
      settings: SourceProductBaseCode=PW,SS
  Solver Configuration : nesl_utility/Solver Configuration  PhysicalDomain=network_engine_domain  SubClassName=solver  LeftPortType=input  RightPortType=generic  Tones=[]  Harmonics=[]  SimulateNoise=off  Profile=off  UseLocalSampling=off  EnableSwitchedLinearOptims=on  FrequencyDomain=off  UseCCode=off  RelTol=0.001  AbsTol=1e-06  MinStep=1e-09  ToWorkspace=off  RevertToSquareIcSolve=off  NumHomotopyIterations=100  PhasorMode=off  PhasorModeNumHarmonics=1  DoDC=off  ResidualTolerance=1e-09  UseLocalSolver=off  LocalSolverChoice=NE_BACKWARD_EULER_ADVANCER  LocalSolverSampleTime=0.001  DoFixedCost=off  MaxNonlinIter=3  MaxModeIter=2  ComputeImpulses=off  ImpulseIterations=2  LinearAlgebra=auto  EquationFormulation=NE_TIME_EF  DelaysMemoryBudget=1024  AutomaticFiltering=on  FilteringTimeConstant=0.001  PartitionStorageMethod=AS_NEEDED  PartitionMemoryBudget=1024  PartitionMethod=ROBUST
      settings: SourceProductBaseCode=PW,SS
  Transform : sm_lib/Frames and Transforms/Rigid Transform  TranslationMethod=Cartesian  TranslationStandardOffset=0  TranslationLengthUnit=mm  TranslationStandardAxis=+Z  TranslationCartesianOffset=smiData.RigidTransform(13).translation  TranslationROffset=0  TranslationROffsetUnits=m  TranslationZOffset=0  TranslationZOffsetUnits=m  TranslationThetaOffset=0  TranslationThetaOffsetUnits=deg  RotationMethod=ArbitraryAxis  RotationAngleUnits=rad  RotationStandardAxis=+Z  RotationAngle=smiData.RigidTransform(13).angle  RotationArbitraryAxis=smiData.RigidTransform(13).axis  FollAlignAxisA=+X  BaseAlignAxisA=+Y  FollAlignAxisB=+Y  BaseAlignAxisB=+Z  RotationSequenceAxes=FollowerAxes  RotationSequence=XYX  RotationSequenceAngles=[0 0 0]  RotationSequenceAnglesUnits=deg  RotationMatrix=[1 0 0; 0 1 0; 0 0 1]
  World : sm_lib/Frames and Transforms/World Frame
  wires:
  psi/1 -> Simulink-PS Converter/1
  theta/1 -> Simulink-PS Converter1/1
  Constant1/1 -> Simulink-PS Converter2/1
  Constant2/1 -> Simulink-PS Converter3/1
  Gain/1 -> Simulink-PS Converter5/1
  Gain1/1 -> Simulink-PS Converter4/1
  thruster_2/1 -> Gain/1
  thruster_1/1 -> Gain1/1
  connections:
  AERO_Fork1_RIGID/RConn1 -- Rotational2/LConn1
  MechanismConfiguration/RConn1 -- Transform/LConn1 -- World/RConn1 -- Solver Configuration/RConn1
  AERO_Propeller1_RIGID/LConn1 -- Rotational5/RConn1
  AERO_Fork1_RIGID/LConn1 -- Rotational1/RConn1
  AERO_Propeller_Housing2_RIGID/LConn1 -- Rotational4/RConn1
  AERO_Arm1_RIGID/RConn2 -- Rotational3/LConn1
  AERO_Propeller_Housing2_RIGID/RConn1 -- Rotational6/LConn1
  AERO_Propeller_Housing1_RIGID/LConn1 -- Rotational3/RConn1
  AERO_Arm1_RIGID/RConn1 -- Rotational4/LConn1
  AERO_Propeller2_RIGID/LConn1 -- Rotational6/RConn1
  Transform/RConn1 -- AERO_Base1_RIGID/LConn1
  AERO_Arm1_RIGID/LConn1 -- Rotational2/RConn1
  AERO_Propeller_Housing1_RIGID/RConn1 -- Rotational5/LConn1
  AERO_Base1_RIGID/RConn1 -- Rotational1/LConn1
  Simulink-PS Converter/RConn1 -- Rotational1/LConn2
  Simulink-PS Converter1/RConn1 -- Rotational2/LConn2
  Simulink-PS Converter2/RConn1 -- Rotational4/LConn2
  Simulink-PS Converter3/RConn1 -- Rotational3/LConn2
  Simulink-PS Converter4/RConn1 -- Rotational5/LConn2
  Simulink-PS Converter5/RConn1 -- Rotational6/LConn2

== system Quanser_AERO_Simulation_2020b/Quanser AERO/Input Noise ==
  u : Inport
  Demux : Demux  Outputs=2
  Motor 0 Noise : simulink/Sources/Band-Limited White Noise  Cov=[noise.motor_0*ts]  Ts=ts  seed=[23341]
  Motor 1 Noise : simulink/Sources/Band-Limited White Noise  Cov=[noise.motor_1*ts]  Ts=ts  seed=[23341]
  Mux : Mux  Inputs=2
  Sum : Sum  Inputs=|++
  Sum1 : Sum  Inputs=++|
  u_noise : Outport  VectorParamsAs1DForOutWhenUnconnected=off
  wires:
  u/1 -> Demux/1
  Demux/2 -> Sum/1
  Demux/1 -> Sum1/2
  Motor 0 Noise/1 -> Sum1/1
  Motor 1 Noise/1 -> Sum/2
  Mux/1 -> u_noise/1
  Sum1/1 -> Mux/1
  Sum/1 -> Mux/2

== system Quanser_AERO_Simulation_2020b/Quanser AERO/Measurement Noise ==
  x : Inport
  Demux : Demux
  Mux : Mux
  Pitch Sensor Noise : simulink/Sources/Band-Limited White Noise  Cov=[noise.pitch*ts]  Ts=ts  seed=[23341]
  Pitch Velocity Sensor Noise : simulink/Sources/Band-Limited White Noise  Cov=[noise.pitch_vel*ts]  Ts=ts  seed=[23341]
  Sum : Sum  Inputs=|++
  Sum1 : Sum  Inputs=|++
  Sum2 : Sum  Inputs=++|
  Sum3 : Sum  Inputs=++|
  Yaw Sensor Noise : simulink/Sources/Band-Limited White Noise  Cov=[noise.yaw*ts]  Ts=ts  seed=[23341]
  Yaw Velocity Sensor Noise : simulink/Sources/Band-Limited White Noise  Cov=[noise.yaw_vel*ts]  Ts=ts  seed=[23341]
  x_noise : Outport  VectorParamsAs1DForOutWhenUnconnected=off
  wires:
  x/1 -> Demux/1
  Demux/3 -> Sum/1
  Demux/4 -> Sum1/1
  Demux/1 -> Sum2/2
  Pitch Sensor Noise/1 -> Sum2/1
  Demux/2 -> Sum3/2
  Pitch Velocity Sensor Noise/1 -> Sum3/1
  Mux/1 -> x_noise/1
  Sum/1 -> Mux/3
  Sum3/1 -> Mux/2
  Sum2/1 -> Mux/1
  Sum1/1 -> Mux/4
  Yaw Sensor Noise/1 -> Sum/2
  Yaw Velocity Sensor Noise/1 -> Sum1/2

== system Quanser_AERO_Simulation_2020b/Quanser AERO/Quanser AERO System Dynamics ==
  x : Inport  OutDataTypeStr=double  PortDimensions=4  SampleTime=0
  u : Inport  Port=2  OutDataTypeStr=double  PortDimensions=2
  model : Inport  Port=3  OutDataTypeStr=double  PortDimensions=1
  MATLAB Function : MATLAB Function  TreatAsAtomicUnit=on
  Saturation : Saturate  UpperLimit=u_lim  LowerLimit=-u_lim
  x_dot : Outport  OutDataTypeStr=double  PortDimensions=4  SampleTime=0  VectorParamsAs1DForOutWhenUnconnected=off
  wires:
  u/1 -> Saturation/1
  MATLAB Function/1(x_dot) -> x_dot/1  "x_dot"
  x/1 -> MATLAB Function/1(x)
  model/1 -> MATLAB Function/3(model)
  Saturation/1 -> MATLAB Function/2(u)
